simulink model "inverted_pendulum"  (R2016a)
settings: Solver=VariableStepAuto  StartTime=0.0  StopTime=10.0  RelTol=1e-3
values from neighbouring files (symbols this model uses):
  g = 9.81    [parameters.m]
  l = 0.5/2    (= 0.25)    [parameters.m]
  M = 0.5    [parameters.m]
  m = 0.1    [parameters.m]
libraries: simulink x2
settings Model: Creator=Duy Nam  LastModifiedBy=Duy Nam

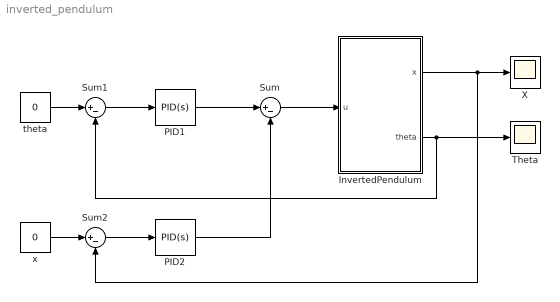
== system inverted_pendulum ==
  "InvertedPendulum " : Subsystem
  "PID1 " : simulink/Continuous/PID Controller  Controller=PID  TimeDomain=Continuous-time  SampleTime=-1  IntegratorMethod=Forward Euler  FilterMethod=Forward Euler  Form=Parallel  UseFilter=on  ControllerParametersSource=internal  P=-30  I=-75  D=-3  N=100  InitialConditionSource=internal  InitialConditionForIntegrator=0  InitialConditionForFilter=0  ExternalReset=none  LimitOutput=off  UpperSaturationLimit=inf  LowerSaturationLimit=-inf  LinearizeAsGain=on  AntiWindupMode=none  Kb=1  TrackingMode=off  Kt=1  PParamMin=[]  PParamMax=[]  IParamMin=[]  IParamMax=[]  DParamMin=[]  DParamMax=[]  NParamMin=[]  NParamMax=[]  KbParamMin=[]  KbParamMax=[]  KtParamMin=[]  KtParamMax=[]  POutMin=[]  POutMax=[]  IOutMin=[]  IOutMax=[]  DOutMin=[]  DOutMax=[]  NOutMin=[]  NOutMax=[]  KbOutMin=[]  KbOutMax=[]  KtOutMin=[]  KtOutMax=[]  IntegratorOutMin=[]  IntegratorOutMax=[]  FilterOutMin=[]  FilterOutMax=[]  SumOutMin=[]  SumOutMax=[]  SumI1OutMin=[]  SumI1OutMax=[]  SumI2OutMin=[]  SumI2OutMax=[]  SumI3OutMin=[]  SumI3OutMax=[]  SumDOutMin=[]  SumDOutMax=[]  SaturationOutMin=[]  SaturationOutMax=[]  IntegratorContinuousStateAttributes=''  IntegratorStateMustResolveToSignalObject=off  IntegratorRTWStateStorageClass=Auto  FilterContinuousStateAttributes=''  FilterStateMustResolveToSignalObject=off  FilterRTWStateStorageClass=Auto  DifferentiatorICPrevScaledInput=0  DifferentiatorOutMin=[]  DifferentiatorOutMax=[]
  PID2 : simulink/Continuous/PID Controller  Controller=PID  TimeDomain=Continuous-time  SampleTime=-1  IntegratorMethod=Forward Euler  FilterMethod=Forward Euler  Form=Parallel  UseFilter=on  ControllerParametersSource=internal  P=-9  I=-5  D=-4  N=100  InitialConditionSource=internal  InitialConditionForIntegrator=0  InitialConditionForFilter=0  ExternalReset=none  LimitOutput=off  UpperSaturationLimit=inf  LowerSaturationLimit=-inf  LinearizeAsGain=on  AntiWindupMode=none  Kb=1  TrackingMode=off  Kt=1  PParamMin=[]  PParamMax=[]  IParamMin=[]  IParamMax=[]  DParamMin=[]  DParamMax=[]  NParamMin=[]  NParamMax=[]  KbParamMin=[]  KbParamMax=[]  KtParamMin=[]  KtParamMax=[]  POutMin=[]  POutMax=[]  IOutMin=[]  IOutMax=[]  DOutMin=[]  DOutMax=[]  NOutMin=[]  NOutMax=[]  KbOutMin=[]  KbOutMax=[]  KtOutMin=[]  KtOutMax=[]  IntegratorOutMin=[]  IntegratorOutMax=[]  FilterOutMin=[]  FilterOutMax=[]  SumOutMin=[]  SumOutMax=[]  SumI1OutMin=[]  SumI1OutMax=[]  SumI2OutMin=[]  SumI2OutMax=[]  SumI3OutMin=[]  SumI3OutMax=[]  SumDOutMin=[]  SumDOutMax=[]  SaturationOutMin=[]  SaturationOutMax=[]  IntegratorContinuousStateAttributes=''  IntegratorStateMustResolveToSignalObject=off  IntegratorRTWStateStorageClass=Auto  FilterContinuousStateAttributes=''  FilterStateMustResolveToSignalObject=off  FilterRTWStateStorageClass=Auto  DifferentiatorICPrevScaledInput=0  DifferentiatorOutMin=[]  DifferentiatorOutMax=[]
  Sum : Sum  Inputs=|+-
  Sum1 : Sum  Inputs=|+-
  Sum2 : Sum  Inputs=|+-
  Theta : Scope
  X : Scope
  theta : Constant  Value=0
  x : Constant  Value=0
  wires:
  Sum2/1 -> PID2/1
  x/1 -> Sum2/1
  Sum1/1 -> "PID1 "/1
  "PID1 "/1 -> Sum/1
  PID2/1 -> Sum/2
  "InvertedPendulum "/1(x) -> Sum2/2, X/1
  "InvertedPendulum "/2(theta) -> Sum1/2, Theta/1
  theta/1 -> Sum1/1
  Sum/1 -> "InvertedPendulum "/1(u)

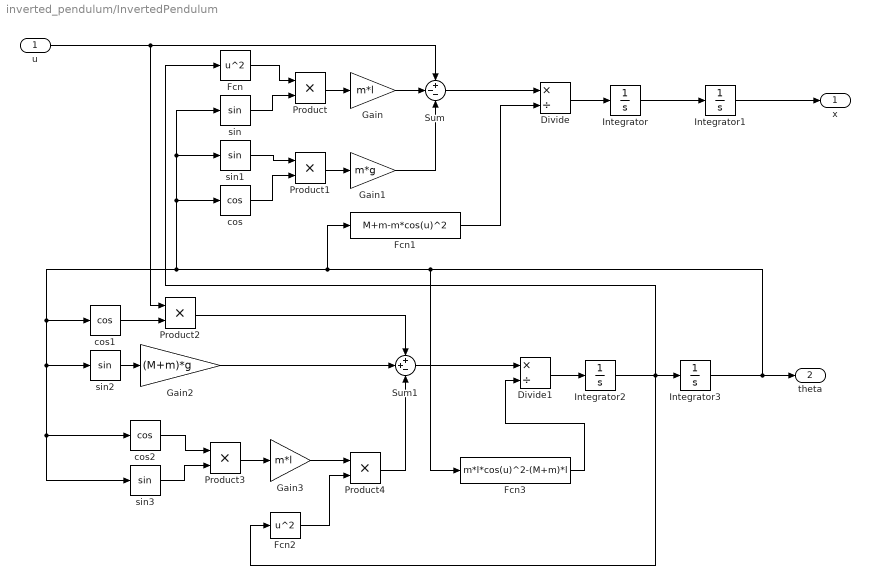
== system inverted_pendulum/InvertedPendulum  ==
  u : Inport
  Divide : Product  Inputs=*/
  Divide1 : Product  Inputs=*/
  Fcn : Fcn  Expr=u^2
  Fcn1 : Fcn  Expr=M+m-m*cos(u)^2
  Fcn2 : Fcn  Expr=u^2
  Fcn3 : Fcn  Expr=m*l*cos(u)^2-(M+m)*l
  Gain : Gain  Gain=m*l
  Gain1 : Gain  Gain=m*g
  Gain2 : Gain  Gain=(M+m)*g
  Gain3 : Gain  Gain=m*l
  Integrator : Integrator
  Integrator1 : Integrator
  Integrator2 : Integrator
  Integrator3 : Integrator  InitialCondition=0.05
  Product{,1..4} (5 alike) : Product
  Sum : Sum  Inputs=+--
  Sum1 : Sum  Inputs=++-
  cos : Trigonometry  Operator=cos
  cos1 : Trigonometry  Operator=cos
  cos2 : Trigonometry  Operator=cos
  sin{,1..3} (4 alike) : Trigonometry
  x : Outport
  theta : Outport  Port=2
  wires:
  Integrator/1 -> Integrator1/1
  Integrator1/1 -> x/1
  Fcn/1 -> Product/1
  sin/1 -> Product/2
  Product/1 -> Gain/1
  u/1 -> Product2/1, Sum/1
  Gain/1 -> Sum/2
  sin1/1 -> Product1/1
  Product1/1 -> Gain1/1
  cos/1 -> Product1/2
  Gain1/1 -> Sum/3
  Integrator2/1 -> Fcn2/1, Fcn/1, Integrator3/1
  Sum/1 -> Divide/1
  Fcn1/1 -> Divide/2
  Divide/1 -> Integrator/1
  cos1/1 -> Product2/2
  sin2/1 -> Gain2/1
  Gain2/1 -> Sum1/2
  Product2/1 -> Sum1/1
  Sum1/1 -> Divide1/1
  Divide1/1 -> Integrator2/1
  Integrator3/1 -> Fcn3/1, sin3/1, cos2/1, sin2/1, cos1/1, cos/1, sin1/1, sin/1, Fcn1/1, theta/1
  cos2/1 -> Product3/1
  sin3/1 -> Product3/2
  Product3/1 -> Gain3/1
  Gain3/1 -> Product4/1
  Fcn2/1 -> Product4/2
  Product4/1 -> Sum1/3
  Fcn3/1 -> Divide1/2
